simulink model "sobelFilter2024a"  (R2024b)
settings: Solver=FixedStepDiscrete  StartTime=0.0  StopTime=2  FixedStep=1/(R*C)  RelTol=1e-3
undefined symbols (not defined in the file or in its folder): gray, R
libraries: hdlsllib x13, visionhdlio x4, visionsources x2
(part 2 of 2)

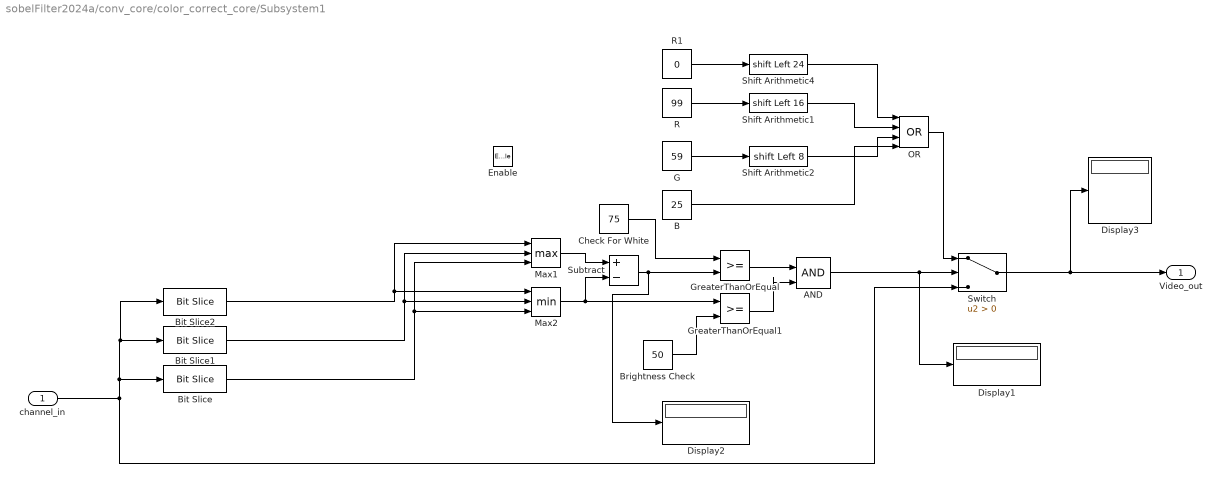
== system sobelFilter2024a/conv_core/color_correct_core/Subsystem1 ==
  channel_in : Inport  OutDataTypeStr=uint32
  Enable : EnablePort
  AND : Logic  IconShape=distinctive  AllPortsSameDT=off  OutDataTypeStr=boolean
  B : Constant  Value=25  OutDataTypeStr=uint8
  Bit Slice : hdlsllib/Logic and Bit Operations/Bit Slice  lidx=7  ridx=0
  Bit Slice1 : hdlsllib/Logic and Bit Operations/Bit Slice  lidx=15  ridx=8
  Bit Slice2 : hdlsllib/Logic and Bit Operations/Bit Slice  lidx=23  ridx=16
  Brightness Check : Constant  Value=50  OutDataTypeStr=uint8
  Check For White : Constant  Value=75  OutDataTypeStr=uint8
  Display1 : Display
      settings: Format=binary (Stored Integer)
  Display2 : Display
      settings: Format=binary (Stored Integer)
  Display3 : Display
      settings: Format=binary (Stored Integer)
  G : Constant  Value=59  OutDataTypeStr=uint8
  GreaterThanOrEqual : RelationalOperator  OutDataTypeStr=boolean  RndMeth=Simplest  InputSameDT=off
  GreaterThanOrEqual1 : RelationalOperator  OutDataTypeStr=boolean  RndMeth=Simplest  InputSameDT=off
  Max1 : MinMax  Function=max  Inputs=3  OutDataTypeStr=uint8
  Max2 : MinMax  Inputs=3  OutDataTypeStr=uint8
  OR : Logic  Operator=OR  Inputs=4  IconShape=distinctive  AllPortsSameDT=off
  R : Constant  Value=99  OutDataTypeStr=uint8
  R1 : Constant  Value=0  OutDataTypeStr=uint8
  Shift Arithmetic1 : ArithShift  BitShiftNumber=16  BitShiftDirection=Left
  Shift Arithmetic2 : ArithShift  BitShiftNumber=8  BitShiftDirection=Left
  Shift Arithmetic4 : ArithShift  BitShiftNumber=24  BitShiftDirection=Left
  Subtract : Sum  Inputs=+-
  Switch : Switch  Criteria=u2 > Threshold  OutDataTypeStr=uint32  SaturateOnIntegerOverflow=off  InputSameDT=off
  Video_out : Outport  OutDataTypeStr=uint32  InitialOutput=[0]
  wires:
  channel_in/1 -> Switch/3, Bit Slice2/1, Bit Slice1/1, Bit Slice/1
  Max1/1 -> Subtract/1
  Max2/1 -> GreaterThanOrEqual1/1, Subtract/2
  Check For White/1 -> GreaterThanOrEqual/1
  GreaterThanOrEqual/1 -> AND/1
  Brightness Check/1 -> GreaterThanOrEqual1/2
  GreaterThanOrEqual1/1 -> AND/2
  Subtract/1 -> GreaterThanOrEqual/2, Display2/1
  AND/1 -> Display1/1, Switch/2
  Switch/1 -> Display3/1, Video_out/1
  Bit Slice2/1 -> Max1/1, Max2/1
  Bit Slice1/1 -> Max2/2, Max1/2
  Bit Slice/1 -> Max2/3, Max1/3
  R1/1 -> Shift Arithmetic4/1
  R/1 -> Shift Arithmetic1/1
  G/1 -> Shift Arithmetic2/1
  B/1 -> OR/4
  Shift Arithmetic2/1 -> OR/3
  Shift Arithmetic1/1 -> OR/2
  Shift Arithmetic4/1 -> OR/1
  OR/1 -> Switch/1

== system sobelFilter2024a/conv_core/gaussian_conv_core/Subsystem1 ==
  note: slice out gray
  channel_in : Inport  OutDataTypeStr=uint8
  coeffs : Inport  Port=2
  Enable : EnablePort
  Delay1 : Delay  DelayLength=1  InitialCondition=0
  Delay2 : Delay  DelayLength=1  InitialCondition=0
  Display : Display
      settings: Format=hex (Stored Integer)
  Mux : Mux  Inputs=9
  Product : Product  SaturateOnIntegerOverflow=on
  Sum of Elements : Sum  Inputs=+  OutDataTypeStr=uint8  SaturateOnIntegerOverflow=on
  slicer : Subsystem
  Video_out : Outport  OutDataTypeStr=uint8  InitialOutput=[0]
  wires:
  slicer/1(out_1) -> Mux/1
  slicer/9(out_9) -> Mux/9
  slicer/5(out_5) -> Mux/5
  slicer/7(out_7) -> Mux/7
  slicer/3(out_3) -> Mux/3
  slicer/6(out_6) -> Mux/6
  slicer/4(out_4) -> Mux/4
  slicer/2(out_2) -> Mux/2
  channel_in/1 -> slicer/1(channel_in)
  slicer/8(out_8) -> Mux/8
  Mux/1 -> Product/2
  coeffs/1 -> Product/1, Display/1
  Product/1 -> Delay1/1
  Delay1/1 -> Sum of Elements/1
  Sum of Elements/1 -> Delay2/1
  Delay2/1 -> Video_out/1

== system sobelFilter2024a/conv_core/just_gray_core/Subsystem1 ==
  note: slice out gray
  note: Grayscale = (R * 0.25) + (G * 0.5) + (B * 0.0625)
  channel_in : Inport  OutDataTypeStr=uint32
  Enable : EnablePort
  Bit Slice1 : hdlsllib/Logic and Bit Operations/Bit Slice  lidx=7  ridx=0
  Bit Slice2 : hdlsllib/Logic and Bit Operations/Bit Slice  lidx=15  ridx=8
  Bit Slice3 : hdlsllib/Logic and Bit Operations/Bit Slice  lidx=23  ridx=16
  Shift Arithmetic3 : ArithShift  BitShiftNumber=1  BitShiftDirection=Right
  Shift Arithmetic4 : ArithShift  BitShiftNumber=2  BitShiftDirection=Right
  Shift Arithmetic5 : ArithShift  BitShiftNumber=4  BitShiftDirection=Right
  Sum : Sum  Inputs=+++  OutDataTypeStr=uint8
  Video_out : Outport  OutDataTypeStr=uint8  InitialOutput=[0]
  wires:
  Shift Arithmetic4/1 -> Sum/1
  Shift Arithmetic3/1 -> Sum/2
  Shift Arithmetic5/1 -> Sum/3
  Bit Slice2/1 -> Shift Arithmetic3/1
  Bit Slice3/1 -> Shift Arithmetic4/1
  channel_in/1 -> Bit Slice3/1, Bit Slice2/1, Bit Slice1/1
  Sum/1 -> Video_out/1
  Bit Slice1/1 -> Shift Arithmetic5/1

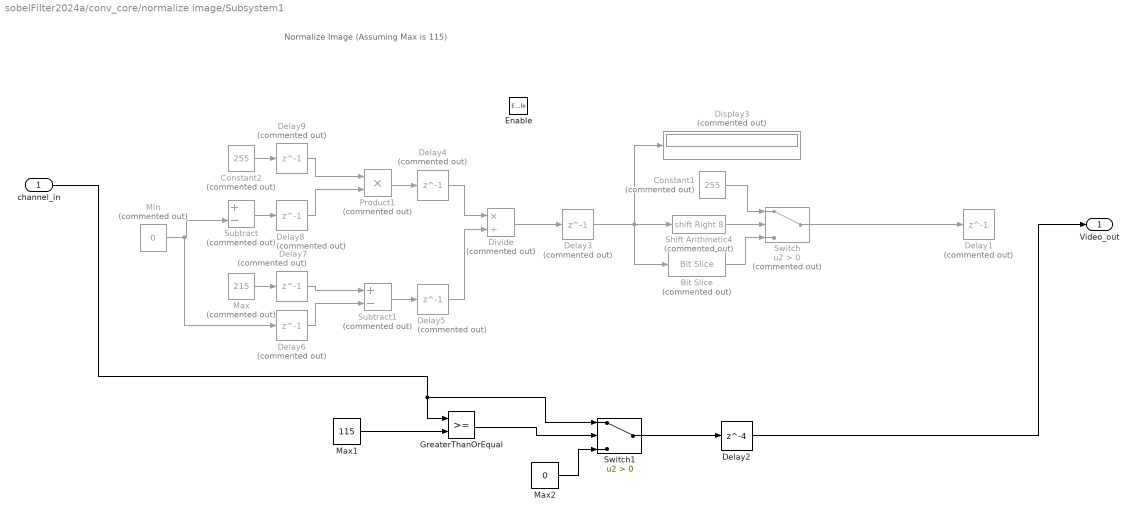
== system sobelFilter2024a/conv_core/normalize image/Subsystem1 ==
  note: Normalize Image (Assuming Max is 115)
  channel_in : Inport  OutDataTypeStr=uint8
  Enable : EnablePort
  Bit Slice : hdlsllib/Logic and Bit Operations/Bit Slice  Commented=on  lidx=7  ridx=0
  Constant1 : Constant  Commented=on  Value=255  OutDataTypeStr=uint8
  Constant2 : Constant  Commented=on  Value=255  OutDataTypeStr=uint8
  Delay{1,3..9} (8 alike) : Delay  Commented=on  DelayLength=1  InitialCondition=0
  Delay2 : Delay  DelayLength=4  InitialCondition=0
  Display3 : Display  Commented=on
      settings: Format=binary (Stored Integer)
  Divide : Product  Commented=on  Inputs=*/
  GreaterThanOrEqual : RelationalOperator  OutDataTypeStr=boolean  RndMeth=Simplest  InputSameDT=off
  Max : Constant  Commented=on  Value=215  OutDataTypeStr=uint8
  Max1 : Constant  Value=115  OutDataTypeStr=uint8
  Max2 : Constant  Value=0  OutDataTypeStr=uint8
  Min : Constant  Commented=on  Value=0  OutDataTypeStr=uint8
  Product1 : Product  Commented=on  SaturateOnIntegerOverflow=on
  Shift Arithmetic4 : ArithShift  Commented=on  BitShiftNumber=8  BitShiftDirection=Right
  Subtract : Sum  Commented=on  Inputs=+-  AccumDataTypeStr=uint8
  Subtract1 : Sum  Commented=on  Inputs=+-  OutDataTypeStr=uint8
  Switch : Switch  Commented=on  Criteria=u2 > Threshold  SaturateOnIntegerOverflow=off  InputSameDT=off
  Switch1 : Switch  Criteria=u2 > Threshold  SaturateOnIntegerOverflow=off  InputSameDT=off
  Video_out : Outport  OutDataTypeStr=uint8  InitialOutput=[0]
  wires:
  Constant2/1 -> Delay9/1
  Subtract/1 -> Delay8/1
  Product1/1 -> Delay4/1
  Max/1 -> Delay7/1
  Min/1 -> Delay6/1, Subtract/2
  Subtract1/1 -> Delay5/1
  Divide/1 -> Delay3/1
  Delay3/1 -> Bit Slice/1, Shift Arithmetic4/1, Display3/1
  Delay4/1 -> Divide/1
  Delay5/1 -> Divide/2
  Delay6/1 -> Subtract1/2
  Delay7/1 -> Subtract1/1
  Delay8/1 -> Product1/2
  Delay9/1 -> Product1/1
  Shift Arithmetic4/1 -> Switch/2
  Switch/1 -> Delay1/1
  Constant1/1 -> Switch/1
  Bit Slice/1 -> Switch/3
  Max1/1 -> GreaterThanOrEqual/2
  channel_in/1 -> Switch1/1, GreaterThanOrEqual/1
  GreaterThanOrEqual/1 -> Switch1/2
  Max2/1 -> Switch1/3
  Switch1/1 -> Delay2/1
  Delay2/1 -> Video_out/1

== system sobelFilter2024a/conv_core/sobel_horz_conv_core/Subsystem1 ==
  note: slice out gray
  channel_in : Inport  OutDataTypeStr=uint8
  coeffs : Inport  Port=2
  Enable : EnablePort
  Delay1 : Delay  DelayLength=1  InitialCondition=0
  Delay2 : Delay  DelayLength=1  InitialCondition=0
  Display : Display
      settings: Format=hex (Stored Integer)
  Mux : Mux  Inputs=9
  Product : Product  SaturateOnIntegerOverflow=on
  Sum of Elements : Sum  Inputs=+  OutDataTypeStr=uint8  SaturateOnIntegerOverflow=on
  slicer : Subsystem
  Video_out : Outport  OutDataTypeStr=uint8  InitialOutput=[0]
  wires:
  slicer/1(out_1) -> Mux/1
  slicer/9(out_9) -> Mux/9
  slicer/5(out_5) -> Mux/5
  slicer/7(out_7) -> Mux/7
  slicer/3(out_3) -> Mux/3
  slicer/6(out_6) -> Mux/6
  slicer/4(out_4) -> Mux/4
  slicer/2(out_2) -> Mux/2
  channel_in/1 -> slicer/1(channel_in)
  slicer/8(out_8) -> Mux/8
  Mux/1 -> Product/2
  coeffs/1 -> Product/1, Display/1
  Product/1 -> Delay1/1
  Delay1/1 -> Sum of Elements/1
  Sum of Elements/1 -> Delay2/1
  Delay2/1 -> Video_out/1

== system sobelFilter2024a/conv_core/sobel_horz_conv_core_alt/Subsystem1 ==
  note: slice out gray
  channel_in : Inport  OutDataTypeStr=uint8
  coeffs : Inport  Port=2
  Enable : EnablePort
  Delay1 : Delay  DelayLength=1  InitialCondition=0
  Delay2 : Delay  DelayLength=1  InitialCondition=0
  Display : Display
      settings: Format=hex (Stored Integer)
  Mux : Mux  Inputs=9
  Product : Product  SaturateOnIntegerOverflow=on
  Sum of Elements : Sum  Inputs=+  OutDataTypeStr=uint8  SaturateOnIntegerOverflow=on
  slicer : Subsystem
  Video_out : Outport  OutDataTypeStr=uint8  InitialOutput=[0]
  wires:
  slicer/1(out_1) -> Mux/1
  slicer/9(out_9) -> Mux/9
  slicer/5(out_5) -> Mux/5
  slicer/7(out_7) -> Mux/7
  slicer/3(out_3) -> Mux/3
  slicer/6(out_6) -> Mux/6
  slicer/4(out_4) -> Mux/4
  slicer/2(out_2) -> Mux/2
  channel_in/1 -> slicer/1(channel_in)
  slicer/8(out_8) -> Mux/8
  Mux/1 -> Product/2
  coeffs/1 -> Product/1, Display/1
  Product/1 -> Delay1/1
  Delay1/1 -> Sum of Elements/1
  Sum of Elements/1 -> Delay2/1
  Delay2/1 -> Video_out/1

== system sobelFilter2024a/conv_core/sobel_vert_conv_core/Subsystem1 ==
  note: slice out gray
  channel_in : Inport  OutDataTypeStr=uint8
  coeffs : Inport  Port=2
  Enable : EnablePort
  Delay1 : Delay  DelayLength=1  InitialCondition=0
  Delay2 : Delay  DelayLength=1  InitialCondition=0
  Display : Display
      settings: Format=hex (Stored Integer)
  Mux : Mux  Inputs=9
  Product : Product  SaturateOnIntegerOverflow=on
  Sum of Elements : Sum  Inputs=+  OutDataTypeStr=uint8  SaturateOnIntegerOverflow=on
  slicer : Subsystem
  Video_out : Outport  OutDataTypeStr=uint8  InitialOutput=[0]
  wires:
  slicer/1(out_1) -> Mux/1
  slicer/9(out_9) -> Mux/9
  slicer/5(out_5) -> Mux/5
  slicer/7(out_7) -> Mux/7
  slicer/3(out_3) -> Mux/3
  slicer/6(out_6) -> Mux/6
  slicer/4(out_4) -> Mux/4
  slicer/2(out_2) -> Mux/2
  channel_in/1 -> slicer/1(channel_in)
  slicer/8(out_8) -> Mux/8
  Mux/1 -> Product/2
  coeffs/1 -> Product/1, Display/1
  Product/1 -> Delay1/1
  Delay1/1 -> Sum of Elements/1
  Sum of Elements/1 -> Delay2/1
  Delay2/1 -> Video_out/1

== system sobelFilter2024a/conv_core/sobel_vert_conv_core_alt/Subsystem1 ==
  note: slice out gray
  channel_in : Inport  OutDataTypeStr=uint8
  coeffs : Inport  Port=2
  Enable : EnablePort
  Delay1 : Delay  DelayLength=1  InitialCondition=0
  Delay2 : Delay  DelayLength=1  InitialCondition=0
  Display : Display
      settings: Format=hex (Stored Integer)
  Mux : Mux  Inputs=9
  Product : Product  SaturateOnIntegerOverflow=on
  Sum of Elements : Sum  Inputs=+  OutDataTypeStr=uint8  SaturateOnIntegerOverflow=on
  slicer : Subsystem
  Video_out : Outport  OutDataTypeStr=uint8  InitialOutput=[0]
  wires:
  slicer/1(out_1) -> Mux/1
  slicer/9(out_9) -> Mux/9
  slicer/5(out_5) -> Mux/5
  slicer/7(out_7) -> Mux/7
  slicer/3(out_3) -> Mux/3
  slicer/6(out_6) -> Mux/6
  slicer/4(out_4) -> Mux/4
  slicer/2(out_2) -> Mux/2
  channel_in/1 -> slicer/1(channel_in)
  slicer/8(out_8) -> Mux/8
  Mux/1 -> Product/2
  coeffs/1 -> Product/1, Display/1
  Product/1 -> Delay1/1
  Delay1/1 -> Sum of Elements/1
  Sum of Elements/1 -> Delay2/1
  Delay2/1 -> Video_out/1

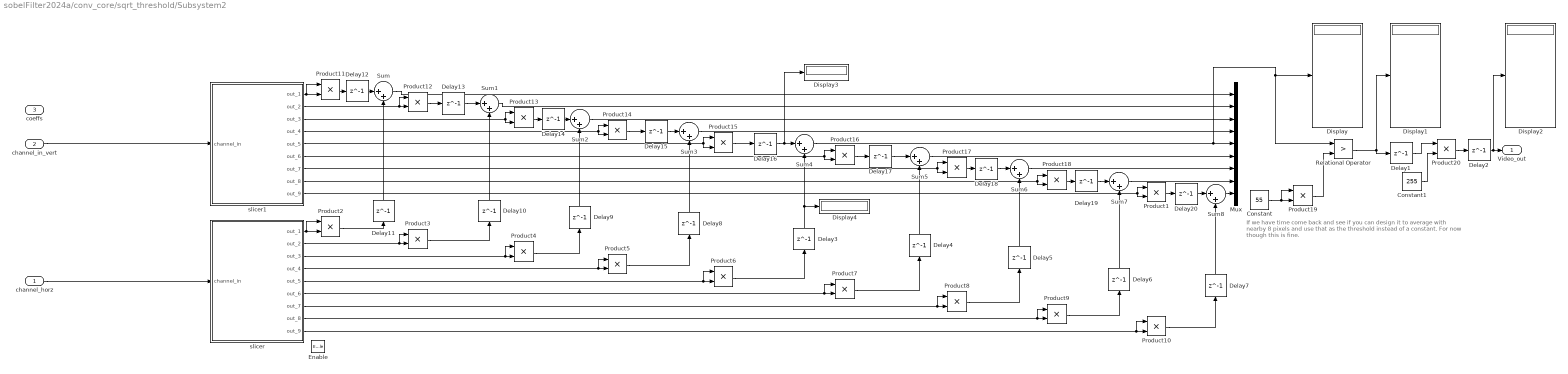
== system sobelFilter2024a/conv_core/sqrt_threshold/Subsystem2 ==
  note: If we have time come back and see if you can design it to average with
      | nearby 8 pixels and use that as the threshold instead of a constant. For
      |  now though this is fine.
  channel_horz : Inport  OutDataTypeStr=uint8
  channel_in_vert : Inport  Port=2
  coeffs : Inport  Port=3
  Enable : EnablePort
  Constant : Constant  Value=55  OutDataTypeStr=uint8
  Constant1 : Constant  Value=255  OutDataTypeStr=uint8
  Delay{1..20} (20 alike) : Delay  DelayLength=1  InitialCondition=0
  Display{,1..4} (5 alike) : Display
      settings: Format=decimal (Stored Integer)
  Mux : Mux  Inputs=9
  Product{1..20} (20 alike) : Product  SaturateOnIntegerOverflow=on
  Relational Operator : RelationalOperator  Operator=>  OutDataTypeStr=boolean  InputSameDT=off
  Sum{,1..8} (9 alike) : Sum  Inputs=|++
  slicer : Subsystem
  slicer1 : Subsystem
  Video_out : Outport  OutDataTypeStr=uint8  InitialOutput=[0]
  wires:
  slicer/1(out_1) -> Product2/1, Product2/2
  slicer/5(out_5) -> Product6/1, Product6/2
  slicer/7(out_7) -> Product8/1, Product8/2
  slicer/3(out_3) -> Product4/1, Product4/2
  slicer/6(out_6) -> Product7/1, Product7/2
  slicer/4(out_4) -> Product5/1, Product5/2
  slicer/2(out_2) -> Product3/1, Product3/2
  channel_horz/1 -> slicer/1(channel_in)
  slicer/8(out_8) -> Product9/1, Product9/2
  Delay2/1 -> Display2/1, Video_out/1
  slicer/9(out_9) -> Product10/1, Product10/2
  slicer1/8(out_8) -> Product18/2, Product18/1
  slicer1/2(out_2) -> Product12/1, Product12/2
  slicer1/9(out_9) -> Product1/2, Product1/1
  slicer1/1(out_1) -> Product11/1, Product11/2
  slicer1/3(out_3) -> Product13/2, Product13/1
  slicer1/7(out_7) -> Product17/2, Product17/1
  slicer1/5(out_5) -> Product15/2, Product15/1
  slicer1/6(out_6) -> Product16/2, Product16/1
  slicer1/4(out_4) -> Product14/2, Product14/1
  channel_in_vert/1 -> slicer1/1(channel_in)
  Product2/1 -> Delay11/1
  Product12/1 -> Delay13/1
  Product3/1 -> Delay10/1
  Product4/1 -> Delay9/1
  Product14/1 -> Delay15/1
  Product5/1 -> Delay8/1
  Product15/1 -> Delay16/1
  Product6/1 -> Delay3/1
  Product16/1 -> Delay17/1
  Product7/1 -> Delay4/1
  Product8/1 -> Delay5/1
  Product9/1 -> Delay6/1
  Product10/1 -> Delay7/1
  Delay1/1 -> Product20/1
  Delay3/1 -> Display4/1, Sum4/2
  Delay4/1 -> Sum5/2
  Delay5/1 -> Sum6/2
  Delay6/1 -> Sum7/2
  Delay7/1 -> Sum8/2
  Delay8/1 -> Sum3/2
  Delay9/1 -> Sum2/2
  Delay10/1 -> Sum1/2
  Delay11/1 -> Sum/2
  Product11/1 -> Delay12/1
  Delay12/1 -> Sum/1
  Delay13/1 -> Sum1/1
  Product13/1 -> Delay14/1
  Delay14/1 -> Sum2/1
  Delay15/1 -> Sum3/1
  Delay16/1 -> Display3/1, Sum4/1
  Delay17/1 -> Sum5/1
  Product17/1 -> Delay18/1
  Delay18/1 -> Sum6/1
  Product18/1 -> Delay19/1
  Delay19/1 -> Sum7/1
  Product1/1 -> Delay20/1
  Delay20/1 -> Sum8/1
  Sum8/1 -> Mux/9
  Sum7/1 -> Mux/8
  Sum6/1 -> Mux/7
  Sum5/1 -> Mux/6
  Sum3/1 -> Mux/4
  Sum2/1 -> Mux/3
  Sum1/1 -> Mux/2
  Sum/1 -> Mux/1
  Constant/1 -> Product19/1, Product19/2
  Product19/1 -> Relational Operator/2
  Relational Operator/1 -> Display1/1, Delay1/1
  Sum4/1 -> Display/1, Relational Operator/1, Mux/5
  Constant1/1 -> Product20/2
  Product20/1 -> Delay2/1

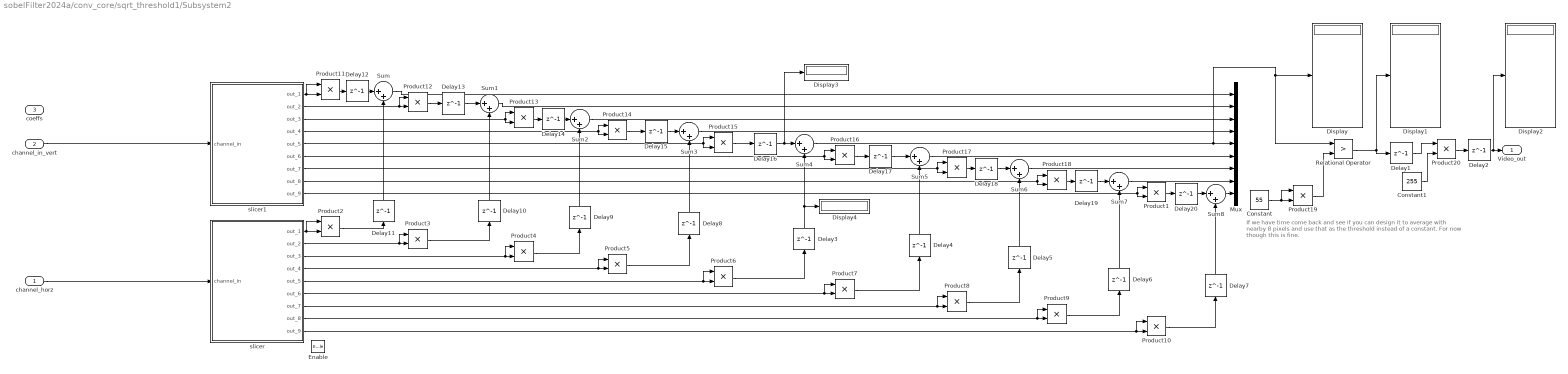
== system sobelFilter2024a/conv_core/sqrt_threshold1/Subsystem2 ==
  note: If we have time come back and see if you can design it to average with
      | nearby 8 pixels and use that as the threshold instead of a constant. For
      |  now though this is fine.
  channel_horz : Inport  OutDataTypeStr=uint8
  channel_in_vert : Inport  Port=2
  coeffs : Inport  Port=3
  Enable : EnablePort
  Constant : Constant  Value=55  OutDataTypeStr=uint8
  Constant1 : Constant  Value=255  OutDataTypeStr=uint8
  Delay{1..20} (20 alike) : Delay  DelayLength=1  InitialCondition=0
  Display{,1..4} (5 alike) : Display
      settings: Format=decimal (Stored Integer)
  Mux : Mux  Inputs=9
  Product{1..20} (20 alike) : Product  SaturateOnIntegerOverflow=on
  Relational Operator : RelationalOperator  Operator=>  OutDataTypeStr=boolean  InputSameDT=off
  Sum{,1..8} (9 alike) : Sum  Inputs=|++
  slicer : Subsystem
  slicer1 : Subsystem
  Video_out : Outport  OutDataTypeStr=uint8  InitialOutput=[0]
  wires:
  slicer/1(out_1) -> Product2/1, Product2/2
  slicer/5(out_5) -> Product6/1, Product6/2
  slicer/7(out_7) -> Product8/1, Product8/2
  slicer/3(out_3) -> Product4/1, Product4/2
  slicer/6(out_6) -> Product7/1, Product7/2
  slicer/4(out_4) -> Product5/1, Product5/2
  slicer/2(out_2) -> Product3/1, Product3/2
  channel_horz/1 -> slicer/1(channel_in)
  slicer/8(out_8) -> Product9/1, Product9/2
  Delay2/1 -> Display2/1, Video_out/1
  slicer/9(out_9) -> Product10/1, Product10/2
  slicer1/8(out_8) -> Product18/2, Product18/1
  slicer1/2(out_2) -> Product12/1, Product12/2
  slicer1/9(out_9) -> Product1/2, Product1/1
  slicer1/1(out_1) -> Product11/1, Product11/2
  slicer1/3(out_3) -> Product13/2, Product13/1
  slicer1/7(out_7) -> Product17/2, Product17/1
  slicer1/5(out_5) -> Product15/2, Product15/1
  slicer1/6(out_6) -> Product16/2, Product16/1
  slicer1/4(out_4) -> Product14/2, Product14/1
  channel_in_vert/1 -> slicer1/1(channel_in)
  Product2/1 -> Delay11/1
  Product12/1 -> Delay13/1
  Product3/1 -> Delay10/1
  Product4/1 -> Delay9/1
  Product14/1 -> Delay15/1
  Product5/1 -> Delay8/1
  Product15/1 -> Delay16/1
  Product6/1 -> Delay3/1
  Product16/1 -> Delay17/1
  Product7/1 -> Delay4/1
  Product8/1 -> Delay5/1
  Product9/1 -> Delay6/1
  Product10/1 -> Delay7/1
  Delay1/1 -> Product20/1
  Delay3/1 -> Display4/1, Sum4/2
  Delay4/1 -> Sum5/2
  Delay5/1 -> Sum6/2
  Delay6/1 -> Sum7/2
  Delay7/1 -> Sum8/2
  Delay8/1 -> Sum3/2
  Delay9/1 -> Sum2/2
  Delay10/1 -> Sum1/2
  Delay11/1 -> Sum/2
  Product11/1 -> Delay12/1
  Delay12/1 -> Sum/1
  Delay13/1 -> Sum1/1
  Product13/1 -> Delay14/1
  Delay14/1 -> Sum2/1
  Delay15/1 -> Sum3/1
  Delay16/1 -> Display3/1, Sum4/1
  Delay17/1 -> Sum5/1
  Product17/1 -> Delay18/1
  Delay18/1 -> Sum6/1
  Product18/1 -> Delay19/1
  Delay19/1 -> Sum7/1
  Product1/1 -> Delay20/1
  Delay20/1 -> Sum8/1
  Sum8/1 -> Mux/9
  Sum7/1 -> Mux/8
  Sum6/1 -> Mux/7
  Sum5/1 -> Mux/6
  Sum3/1 -> Mux/4
  Sum2/1 -> Mux/3
  Sum1/1 -> Mux/2
  Sum/1 -> Mux/1
  Constant/1 -> Product19/1, Product19/2
  Product19/1 -> Relational Operator/2
  Relational Operator/1 -> Display1/1, Delay1/1
  Sum4/1 -> Display/1, Relational Operator/1, Mux/5
  Constant1/1 -> Product20/2
  Product20/1 -> Delay2/1

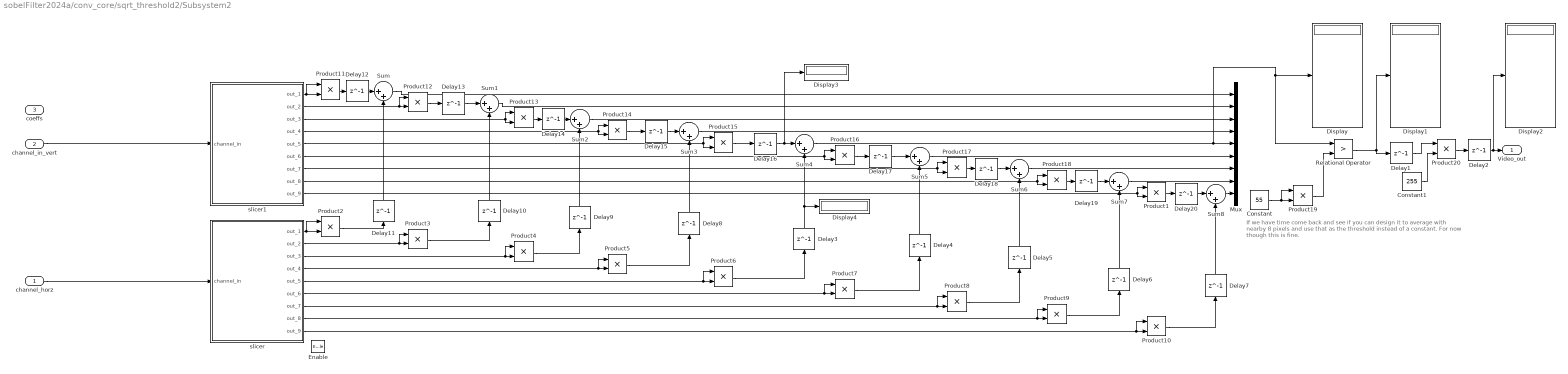
== system sobelFilter2024a/conv_core/sqrt_threshold2/Subsystem2 ==
  note: If we have time come back and see if you can design it to average with
      | nearby 8 pixels and use that as the threshold instead of a constant. For
      |  now though this is fine.
  channel_horz : Inport  OutDataTypeStr=uint8
  channel_in_vert : Inport  Port=2
  coeffs : Inport  Port=3
  Enable : EnablePort
  Constant : Constant  Value=55  OutDataTypeStr=uint8
  Constant1 : Constant  Value=255  OutDataTypeStr=uint8
  Delay{1..20} (20 alike) : Delay  DelayLength=1  InitialCondition=0
  Display{,1..4} (5 alike) : Display
      settings: Format=decimal (Stored Integer)
  Mux : Mux  Inputs=9
  Product{1..20} (20 alike) : Product  SaturateOnIntegerOverflow=on
  Relational Operator : RelationalOperator  Operator=>  OutDataTypeStr=boolean  InputSameDT=off
  Sum{,1..8} (9 alike) : Sum  Inputs=|++
  slicer : Subsystem
  slicer1 : Subsystem
  Video_out : Outport  OutDataTypeStr=uint8  InitialOutput=[0]
  wires:
  slicer/1(out_1) -> Product2/1, Product2/2
  slicer/5(out_5) -> Product6/1, Product6/2
  slicer/7(out_7) -> Product8/1, Product8/2
  slicer/3(out_3) -> Product4/1, Product4/2
  slicer/6(out_6) -> Product7/1, Product7/2
  slicer/4(out_4) -> Product5/1, Product5/2
  slicer/2(out_2) -> Product3/1, Product3/2
  channel_horz/1 -> slicer/1(channel_in)
  slicer/8(out_8) -> Product9/1, Product9/2
  Delay2/1 -> Display2/1, Video_out/1
  slicer/9(out_9) -> Product10/1, Product10/2
  slicer1/8(out_8) -> Product18/2, Product18/1
  slicer1/2(out_2) -> Product12/1, Product12/2
  slicer1/9(out_9) -> Product1/2, Product1/1
  slicer1/1(out_1) -> Product11/1, Product11/2
  slicer1/3(out_3) -> Product13/2, Product13/1
  slicer1/7(out_7) -> Product17/2, Product17/1
  slicer1/5(out_5) -> Product15/2, Product15/1
  slicer1/6(out_6) -> Product16/2, Product16/1
  slicer1/4(out_4) -> Product14/2, Product14/1
  channel_in_vert/1 -> slicer1/1(channel_in)
  Product2/1 -> Delay11/1
  Product12/1 -> Delay13/1
  Product3/1 -> Delay10/1
  Product4/1 -> Delay9/1
  Product14/1 -> Delay15/1
  Product5/1 -> Delay8/1
  Product15/1 -> Delay16/1
  Product6/1 -> Delay3/1
  Product16/1 -> Delay17/1
  Product7/1 -> Delay4/1
  Product8/1 -> Delay5/1
  Product9/1 -> Delay6/1
  Product10/1 -> Delay7/1
  Delay1/1 -> Product20/1
  Delay3/1 -> Display4/1, Sum4/2
  Delay4/1 -> Sum5/2
  Delay5/1 -> Sum6/2
  Delay6/1 -> Sum7/2
  Delay7/1 -> Sum8/2
  Delay8/1 -> Sum3/2
  Delay9/1 -> Sum2/2
  Delay10/1 -> Sum1/2
  Delay11/1 -> Sum/2
  Product11/1 -> Delay12/1
  Delay12/1 -> Sum/1
  Delay13/1 -> Sum1/1
  Product13/1 -> Delay14/1
  Delay14/1 -> Sum2/1
  Delay15/1 -> Sum3/1
  Delay16/1 -> Display3/1, Sum4/1
  Delay17/1 -> Sum5/1
  Product17/1 -> Delay18/1
  Delay18/1 -> Sum6/1
  Product18/1 -> Delay19/1
  Delay19/1 -> Sum7/1
  Product1/1 -> Delay20/1
  Delay20/1 -> Sum8/1
  Sum8/1 -> Mux/9
  Sum7/1 -> Mux/8
  Sum6/1 -> Mux/7
  Sum5/1 -> Mux/6
  Sum3/1 -> Mux/4
  Sum2/1 -> Mux/3
  Sum1/1 -> Mux/2
  Sum/1 -> Mux/1
  Constant/1 -> Product19/1, Product19/2
  Product19/1 -> Relational Operator/2
  Relational Operator/1 -> Display1/1, Delay1/1
  Sum4/1 -> Display/1, Relational Operator/1, Mux/5
  Constant1/1 -> Product20/2
  Product20/1 -> Delay2/1

== system sobelFilter2024a/gaussian_conv_core/Subsystem1/slicer ==
  channel_in : Inport
  Delay{1..6} (6 alike) : Delay  DelayLength=1  InitialCondition=0
  Line buffer : Delay  DelayLength=R-2  InitialCondition=0
  Line buffer1 : Delay  DelayLength=R-2  InitialCondition=0
  out_1 : Outport  VectorParamsAs1DForOutWhenUnconnected=off
  out_2 : Outport  Port=2  VectorParamsAs1DForOutWhenUnconnected=off
  out_3 : Outport  Port=3  VectorParamsAs1DForOutWhenUnconnected=off
  out_4 : Outport  Port=4  VectorParamsAs1DForOutWhenUnconnected=off
  out_5 : Outport  Port=5  VectorParamsAs1DForOutWhenUnconnected=off
  out_6 : Outport  Port=6  VectorParamsAs1DForOutWhenUnconnected=off
  out_7 : Outport  Port=7  VectorParamsAs1DForOutWhenUnconnected=off
  out_8 : Outport  Port=8  VectorParamsAs1DForOutWhenUnconnected=off
  out_9 : Outport  Port=9  VectorParamsAs1DForOutWhenUnconnected=off
  wires:
  Delay4/1 -> Line buffer/1, out_3/1
  channel_in/1 -> out_1/1, Delay1/1
  Delay1/1 -> out_2/1, Delay4/1
  Delay3/1 -> out_8/1, Delay6/1
  Delay5/1 -> Line buffer1/1, out_6/1
  Delay6/1 -> out_9/1
  Line buffer/1 -> out_4/1, Delay2/1
  Line buffer1/1 -> out_7/1, Delay3/1
  Delay2/1 -> out_5/1, Delay5/1

== system sobelFilter2024a/sobel_horz_conv_core/Subsystem1/slicer ==
  channel_in : Inport
  Delay{1..6} (6 alike) : Delay  DelayLength=1  InitialCondition=0
  Line buffer : Delay  DelayLength=R-2  InitialCondition=0
  Line buffer1 : Delay  DelayLength=R-2  InitialCondition=0
  out_1 : Outport  VectorParamsAs1DForOutWhenUnconnected=off
  out_2 : Outport  Port=2  VectorParamsAs1DForOutWhenUnconnected=off
  out_3 : Outport  Port=3  VectorParamsAs1DForOutWhenUnconnected=off
  out_4 : Outport  Port=4  VectorParamsAs1DForOutWhenUnconnected=off
  out_5 : Outport  Port=5  VectorParamsAs1DForOutWhenUnconnected=off
  out_6 : Outport  Port=6  VectorParamsAs1DForOutWhenUnconnected=off
  out_7 : Outport  Port=7  VectorParamsAs1DForOutWhenUnconnected=off
  out_8 : Outport  Port=8  VectorParamsAs1DForOutWhenUnconnected=off
  out_9 : Outport  Port=9  VectorParamsAs1DForOutWhenUnconnected=off
  wires:
  Delay4/1 -> Line buffer/1, out_3/1
  channel_in/1 -> out_1/1, Delay1/1
  Delay1/1 -> out_2/1, Delay4/1
  Delay3/1 -> out_8/1, Delay6/1
  Delay5/1 -> Line buffer1/1, out_6/1
  Delay6/1 -> out_9/1
  Line buffer/1 -> out_4/1, Delay2/1
  Line buffer1/1 -> out_7/1, Delay3/1
  Delay2/1 -> out_5/1, Delay5/1

== system sobelFilter2024a/sobel_horz_conv_core_alt/Subsystem1/slicer ==
  channel_in : Inport
  Delay{1..6} (6 alike) : Delay  DelayLength=1  InitialCondition=0
  Line buffer : Delay  DelayLength=R-2  InitialCondition=0
  Line buffer1 : Delay  DelayLength=R-2  InitialCondition=0
  out_1 : Outport  VectorParamsAs1DForOutWhenUnconnected=off
  out_2 : Outport  Port=2  VectorParamsAs1DForOutWhenUnconnected=off
  out_3 : Outport  Port=3  VectorParamsAs1DForOutWhenUnconnected=off
  out_4 : Outport  Port=4  VectorParamsAs1DForOutWhenUnconnected=off
  out_5 : Outport  Port=5  VectorParamsAs1DForOutWhenUnconnected=off
  out_6 : Outport  Port=6  VectorParamsAs1DForOutWhenUnconnected=off
  out_7 : Outport  Port=7  VectorParamsAs1DForOutWhenUnconnected=off
  out_8 : Outport  Port=8  VectorParamsAs1DForOutWhenUnconnected=off
  out_9 : Outport  Port=9  VectorParamsAs1DForOutWhenUnconnected=off
  wires:
  Delay4/1 -> Line buffer/1, out_3/1
  channel_in/1 -> out_1/1, Delay1/1
  Delay1/1 -> out_2/1, Delay4/1
  Delay3/1 -> out_8/1, Delay6/1
  Delay5/1 -> Line buffer1/1, out_6/1
  Delay6/1 -> out_9/1
  Line buffer/1 -> out_4/1, Delay2/1
  Line buffer1/1 -> out_7/1, Delay3/1
  Delay2/1 -> out_5/1, Delay5/1

== system sobelFilter2024a/sobel_vert_conv_core/Subsystem1/slicer ==
  channel_in : Inport
  Delay{1..6} (6 alike) : Delay  DelayLength=1  InitialCondition=0
  Line buffer : Delay  DelayLength=R-2  InitialCondition=0
  Line buffer1 : Delay  DelayLength=R-2  InitialCondition=0
  out_1 : Outport  VectorParamsAs1DForOutWhenUnconnected=off
  out_2 : Outport  Port=2  VectorParamsAs1DForOutWhenUnconnected=off
  out_3 : Outport  Port=3  VectorParamsAs1DForOutWhenUnconnected=off
  out_4 : Outport  Port=4  VectorParamsAs1DForOutWhenUnconnected=off
  out_5 : Outport  Port=5  VectorParamsAs1DForOutWhenUnconnected=off
  out_6 : Outport  Port=6  VectorParamsAs1DForOutWhenUnconnected=off
  out_7 : Outport  Port=7  VectorParamsAs1DForOutWhenUnconnected=off
  out_8 : Outport  Port=8  VectorParamsAs1DForOutWhenUnconnected=off
  out_9 : Outport  Port=9  VectorParamsAs1DForOutWhenUnconnected=off
  wires:
  Delay4/1 -> Line buffer/1, out_3/1
  channel_in/1 -> out_1/1, Delay1/1
  Delay1/1 -> out_2/1, Delay4/1
  Delay3/1 -> out_8/1, Delay6/1
  Delay5/1 -> Line buffer1/1, out_6/1
  Delay6/1 -> out_9/1
  Line buffer/1 -> out_4/1, Delay2/1
  Line buffer1/1 -> out_7/1, Delay3/1
  Delay2/1 -> out_5/1, Delay5/1

== system sobelFilter2024a/sobel_vert_conv_core_alt/Subsystem1/slicer ==
  channel_in : Inport
  Delay{1..6} (6 alike) : Delay  DelayLength=1  InitialCondition=0
  Line buffer : Delay  DelayLength=R-2  InitialCondition=0
  Line buffer1 : Delay  DelayLength=R-2  InitialCondition=0
  out_1 : Outport  VectorParamsAs1DForOutWhenUnconnected=off
  out_2 : Outport  Port=2  VectorParamsAs1DForOutWhenUnconnected=off
  out_3 : Outport  Port=3  VectorParamsAs1DForOutWhenUnconnected=off
  out_4 : Outport  Port=4  VectorParamsAs1DForOutWhenUnconnected=off
  out_5 : Outport  Port=5  VectorParamsAs1DForOutWhenUnconnected=off
  out_6 : Outport  Port=6  VectorParamsAs1DForOutWhenUnconnected=off
  out_7 : Outport  Port=7  VectorParamsAs1DForOutWhenUnconnected=off
  out_8 : Outport  Port=8  VectorParamsAs1DForOutWhenUnconnected=off
  out_9 : Outport  Port=9  VectorParamsAs1DForOutWhenUnconnected=off
  wires:
  Delay4/1 -> Line buffer/1, out_3/1
  channel_in/1 -> out_1/1, Delay1/1
  Delay1/1 -> out_2/1, Delay4/1
  Delay3/1 -> out_8/1, Delay6/1
  Delay5/1 -> Line buffer1/1, out_6/1
  Delay6/1 -> out_9/1
  Line buffer/1 -> out_4/1, Delay2/1
  Line buffer1/1 -> out_7/1, Delay3/1
  Delay2/1 -> out_5/1, Delay5/1

== system sobelFilter2024a/sqrt_threshold/Subsystem2/slicer ==
  channel_in : Inport
  Delay{1..6} (6 alike) : Delay  DelayLength=1  InitialCondition=0
  Line buffer : Delay  DelayLength=R-2  InitialCondition=0
  Line buffer1 : Delay  DelayLength=R-2  InitialCondition=0
  out_1 : Outport  VectorParamsAs1DForOutWhenUnconnected=off
  out_2 : Outport  Port=2  VectorParamsAs1DForOutWhenUnconnected=off
  out_3 : Outport  Port=3  VectorParamsAs1DForOutWhenUnconnected=off
  out_4 : Outport  Port=4  VectorParamsAs1DForOutWhenUnconnected=off
  out_5 : Outport  Port=5  VectorParamsAs1DForOutWhenUnconnected=off
  out_6 : Outport  Port=6  VectorParamsAs1DForOutWhenUnconnected=off
  out_7 : Outport  Port=7  VectorParamsAs1DForOutWhenUnconnected=off
  out_8 : Outport  Port=8  VectorParamsAs1DForOutWhenUnconnected=off
  out_9 : Outport  Port=9  VectorParamsAs1DForOutWhenUnconnected=off
  wires:
  Delay4/1 -> Line buffer/1, out_3/1
  channel_in/1 -> out_1/1, Delay1/1
  Delay1/1 -> out_2/1, Delay4/1
  Delay3/1 -> out_8/1, Delay6/1
  Delay5/1 -> Line buffer1/1, out_6/1
  Delay6/1 -> out_9/1
  Line buffer/1 -> out_4/1, Delay2/1
  Line buffer1/1 -> out_7/1, Delay3/1
  Delay2/1 -> out_5/1, Delay5/1

== system sobelFilter2024a/sqrt_threshold/Subsystem2/slicer1 ==
  channel_in : Inport
  Delay{1..6} (6 alike) : Delay  DelayLength=1  InitialCondition=0
  Line buffer : Delay  DelayLength=R-2  InitialCondition=0
  Line buffer1 : Delay  DelayLength=R-2  InitialCondition=0
  out_1 : Outport  VectorParamsAs1DForOutWhenUnconnected=off
  out_2 : Outport  Port=2  VectorParamsAs1DForOutWhenUnconnected=off
  out_3 : Outport  Port=3  VectorParamsAs1DForOutWhenUnconnected=off
  out_4 : Outport  Port=4  VectorParamsAs1DForOutWhenUnconnected=off
  out_5 : Outport  Port=5  VectorParamsAs1DForOutWhenUnconnected=off
  out_6 : Outport  Port=6  VectorParamsAs1DForOutWhenUnconnected=off
  out_7 : Outport  Port=7  VectorParamsAs1DForOutWhenUnconnected=off
  out_8 : Outport  Port=8  VectorParamsAs1DForOutWhenUnconnected=off
  out_9 : Outport  Port=9  VectorParamsAs1DForOutWhenUnconnected=off
  wires:
  Delay4/1 -> Line buffer/1, out_3/1
  channel_in/1 -> out_1/1, Delay1/1
  Delay1/1 -> out_2/1, Delay4/1
  Delay3/1 -> out_8/1, Delay6/1
  Delay5/1 -> Line buffer1/1, out_6/1
  Delay6/1 -> out_9/1
  Line buffer/1 -> out_4/1, Delay2/1
  Line buffer1/1 -> out_7/1, Delay3/1
  Delay2/1 -> out_5/1, Delay5/1

== system sobelFilter2024a/sqrt_threshold1/Subsystem2/slicer ==
  channel_in : Inport
  Delay{1..6} (6 alike) : Delay  DelayLength=1  InitialCondition=0
  Line buffer : Delay  DelayLength=R-2  InitialCondition=0
  Line buffer1 : Delay  DelayLength=R-2  InitialCondition=0
  out_1 : Outport  VectorParamsAs1DForOutWhenUnconnected=off
  out_2 : Outport  Port=2  VectorParamsAs1DForOutWhenUnconnected=off
  out_3 : Outport  Port=3  VectorParamsAs1DForOutWhenUnconnected=off
  out_4 : Outport  Port=4  VectorParamsAs1DForOutWhenUnconnected=off
  out_5 : Outport  Port=5  VectorParamsAs1DForOutWhenUnconnected=off
  out_6 : Outport  Port=6  VectorParamsAs1DForOutWhenUnconnected=off
  out_7 : Outport  Port=7  VectorParamsAs1DForOutWhenUnconnected=off
  out_8 : Outport  Port=8  VectorParamsAs1DForOutWhenUnconnected=off
  out_9 : Outport  Port=9  VectorParamsAs1DForOutWhenUnconnected=off
  wires:
  Delay4/1 -> Line buffer/1, out_3/1
  channel_in/1 -> out_1/1, Delay1/1
  Delay1/1 -> out_2/1, Delay4/1
  Delay3/1 -> out_8/1, Delay6/1
  Delay5/1 -> Line buffer1/1, out_6/1
  Delay6/1 -> out_9/1
  Line buffer/1 -> out_4/1, Delay2/1
  Line buffer1/1 -> out_7/1, Delay3/1
  Delay2/1 -> out_5/1, Delay5/1

== system sobelFilter2024a/sqrt_threshold1/Subsystem2/slicer1 ==
  channel_in : Inport
  Delay{1..6} (6 alike) : Delay  DelayLength=1  InitialCondition=0
  Line buffer : Delay  DelayLength=R-2  InitialCondition=0
  Line buffer1 : Delay  DelayLength=R-2  InitialCondition=0
  out_1 : Outport  VectorParamsAs1DForOutWhenUnconnected=off
  out_2 : Outport  Port=2  VectorParamsAs1DForOutWhenUnconnected=off
  out_3 : Outport  Port=3  VectorParamsAs1DForOutWhenUnconnected=off
  out_4 : Outport  Port=4  VectorParamsAs1DForOutWhenUnconnected=off
  out_5 : Outport  Port=5  VectorParamsAs1DForOutWhenUnconnected=off
  out_6 : Outport  Port=6  VectorParamsAs1DForOutWhenUnconnected=off
  out_7 : Outport  Port=7  VectorParamsAs1DForOutWhenUnconnected=off
  out_8 : Outport  Port=8  VectorParamsAs1DForOutWhenUnconnected=off
  out_9 : Outport  Port=9  VectorParamsAs1DForOutWhenUnconnected=off
  wires:
  Delay4/1 -> Line buffer/1, out_3/1
  channel_in/1 -> out_1/1, Delay1/1
  Delay1/1 -> out_2/1, Delay4/1
  Delay3/1 -> out_8/1, Delay6/1
  Delay5/1 -> Line buffer1/1, out_6/1
  Delay6/1 -> out_9/1
  Line buffer/1 -> out_4/1, Delay2/1
  Line buffer1/1 -> out_7/1, Delay3/1
  Delay2/1 -> out_5/1, Delay5/1

== system sobelFilter2024a/sqrt_threshold2/Subsystem2/slicer ==
  channel_in : Inport
  Delay{1..6} (6 alike) : Delay  DelayLength=1  InitialCondition=0
  Line buffer : Delay  DelayLength=R-2  InitialCondition=0
  Line buffer1 : Delay  DelayLength=R-2  InitialCondition=0
  out_1 : Outport  VectorParamsAs1DForOutWhenUnconnected=off
  out_2 : Outport  Port=2  VectorParamsAs1DForOutWhenUnconnected=off
  out_3 : Outport  Port=3  VectorParamsAs1DForOutWhenUnconnected=off
  out_4 : Outport  Port=4  VectorParamsAs1DForOutWhenUnconnected=off
  out_5 : Outport  Port=5  VectorParamsAs1DForOutWhenUnconnected=off
  out_6 : Outport  Port=6  VectorParamsAs1DForOutWhenUnconnected=off
  out_7 : Outport  Port=7  VectorParamsAs1DForOutWhenUnconnected=off
  out_8 : Outport  Port=8  VectorParamsAs1DForOutWhenUnconnected=off
  out_9 : Outport  Port=9  VectorParamsAs1DForOutWhenUnconnected=off
  wires:
  Delay4/1 -> Line buffer/1, out_3/1
  channel_in/1 -> out_1/1, Delay1/1
  Delay1/1 -> out_2/1, Delay4/1
  Delay3/1 -> out_8/1, Delay6/1
  Delay5/1 -> Line buffer1/1, out_6/1
  Delay6/1 -> out_9/1
  Line buffer/1 -> out_4/1, Delay2/1
  Line buffer1/1 -> out_7/1, Delay3/1
  Delay2/1 -> out_5/1, Delay5/1

== system sobelFilter2024a/sqrt_threshold2/Subsystem2/slicer1 ==
  channel_in : Inport
  Delay{1..6} (6 alike) : Delay  DelayLength=1  InitialCondition=0
  Line buffer : Delay  DelayLength=R-2  InitialCondition=0
  Line buffer1 : Delay  DelayLength=R-2  InitialCondition=0
  out_1 : Outport  VectorParamsAs1DForOutWhenUnconnected=off
  out_2 : Outport  Port=2  VectorParamsAs1DForOutWhenUnconnected=off
  out_3 : Outport  Port=3  VectorParamsAs1DForOutWhenUnconnected=off
  out_4 : Outport  Port=4  VectorParamsAs1DForOutWhenUnconnected=off
  out_5 : Outport  Port=5  VectorParamsAs1DForOutWhenUnconnected=off
  out_6 : Outport  Port=6  VectorParamsAs1DForOutWhenUnconnected=off
  out_7 : Outport  Port=7  VectorParamsAs1DForOutWhenUnconnected=off
  out_8 : Outport  Port=8  VectorParamsAs1DForOutWhenUnconnected=off
  out_9 : Outport  Port=9  VectorParamsAs1DForOutWhenUnconnected=off
  wires:
  Delay4/1 -> Line buffer/1, out_3/1
  channel_in/1 -> out_1/1, Delay1/1
  Delay1/1 -> out_2/1, Delay4/1
  Delay3/1 -> out_8/1, Delay6/1
  Delay5/1 -> Line buffer1/1, out_6/1
  Delay6/1 -> out_9/1
  Line buffer/1 -> out_4/1, Delay2/1
  Line buffer1/1 -> out_7/1, Delay3/1
  Delay2/1 -> out_5/1, Delay5/1

== system sobelFilter2024a/conv_core/gaussian_conv_core/Subsystem1/slicer ==
  channel_in : Inport
  Delay{1..6} (6 alike) : Delay  DelayLength=1  InitialCondition=0
  Line buffer : Delay  DelayLength=R-2  InitialCondition=0
  Line buffer1 : Delay  DelayLength=R-2  InitialCondition=0
  out_1 : Outport  VectorParamsAs1DForOutWhenUnconnected=off
  out_2 : Outport  Port=2  VectorParamsAs1DForOutWhenUnconnected=off
  out_3 : Outport  Port=3  VectorParamsAs1DForOutWhenUnconnected=off
  out_4 : Outport  Port=4  VectorParamsAs1DForOutWhenUnconnected=off
  out_5 : Outport  Port=5  VectorParamsAs1DForOutWhenUnconnected=off
  out_6 : Outport  Port=6  VectorParamsAs1DForOutWhenUnconnected=off
  out_7 : Outport  Port=7  VectorParamsAs1DForOutWhenUnconnected=off
  out_8 : Outport  Port=8  VectorParamsAs1DForOutWhenUnconnected=off
  out_9 : Outport  Port=9  VectorParamsAs1DForOutWhenUnconnected=off
  wires:
  Delay4/1 -> Line buffer/1, out_3/1
  channel_in/1 -> out_1/1, Delay1/1
  Delay1/1 -> out_2/1, Delay4/1
  Delay3/1 -> out_8/1, Delay6/1
  Delay5/1 -> Line buffer1/1, out_6/1
  Delay6/1 -> out_9/1
  Line buffer/1 -> out_4/1, Delay2/1
  Line buffer1/1 -> out_7/1, Delay3/1
  Delay2/1 -> out_5/1, Delay5/1

== system sobelFilter2024a/conv_core/sobel_horz_conv_core/Subsystem1/slicer ==
  channel_in : Inport
  Delay{1..6} (6 alike) : Delay  DelayLength=1  InitialCondition=0
  Line buffer : Delay  DelayLength=R-2  InitialCondition=0
  Line buffer1 : Delay  DelayLength=R-2  InitialCondition=0
  out_1 : Outport  VectorParamsAs1DForOutWhenUnconnected=off
  out_2 : Outport  Port=2  VectorParamsAs1DForOutWhenUnconnected=off
  out_3 : Outport  Port=3  VectorParamsAs1DForOutWhenUnconnected=off
  out_4 : Outport  Port=4  VectorParamsAs1DForOutWhenUnconnected=off
  out_5 : Outport  Port=5  VectorParamsAs1DForOutWhenUnconnected=off
  out_6 : Outport  Port=6  VectorParamsAs1DForOutWhenUnconnected=off
  out_7 : Outport  Port=7  VectorParamsAs1DForOutWhenUnconnected=off
  out_8 : Outport  Port=8  VectorParamsAs1DForOutWhenUnconnected=off
  out_9 : Outport  Port=9  VectorParamsAs1DForOutWhenUnconnected=off
  wires:
  Delay4/1 -> Line buffer/1, out_3/1
  channel_in/1 -> out_1/1, Delay1/1
  Delay1/1 -> out_2/1, Delay4/1
  Delay3/1 -> out_8/1, Delay6/1
  Delay5/1 -> Line buffer1/1, out_6/1
  Delay6/1 -> out_9/1
  Line buffer/1 -> out_4/1, Delay2/1
  Line buffer1/1 -> out_7/1, Delay3/1
  Delay2/1 -> out_5/1, Delay5/1

== system sobelFilter2024a/conv_core/sobel_horz_conv_core_alt/Subsystem1/slicer ==
  channel_in : Inport
  Delay{1..6} (6 alike) : Delay  DelayLength=1  InitialCondition=0
  Line buffer : Delay  DelayLength=R-2  InitialCondition=0
  Line buffer1 : Delay  DelayLength=R-2  InitialCondition=0
  out_1 : Outport  VectorParamsAs1DForOutWhenUnconnected=off
  out_2 : Outport  Port=2  VectorParamsAs1DForOutWhenUnconnected=off
  out_3 : Outport  Port=3  VectorParamsAs1DForOutWhenUnconnected=off
  out_4 : Outport  Port=4  VectorParamsAs1DForOutWhenUnconnected=off
  out_5 : Outport  Port=5  VectorParamsAs1DForOutWhenUnconnected=off
  out_6 : Outport  Port=6  VectorParamsAs1DForOutWhenUnconnected=off
  out_7 : Outport  Port=7  VectorParamsAs1DForOutWhenUnconnected=off
  out_8 : Outport  Port=8  VectorParamsAs1DForOutWhenUnconnected=off
  out_9 : Outport  Port=9  VectorParamsAs1DForOutWhenUnconnected=off
  wires:
  Delay4/1 -> Line buffer/1, out_3/1
  channel_in/1 -> out_1/1, Delay1/1
  Delay1/1 -> out_2/1, Delay4/1
  Delay3/1 -> out_8/1, Delay6/1
  Delay5/1 -> Line buffer1/1, out_6/1
  Delay6/1 -> out_9/1
  Line buffer/1 -> out_4/1, Delay2/1
  Line buffer1/1 -> out_7/1, Delay3/1
  Delay2/1 -> out_5/1, Delay5/1

== system sobelFilter2024a/conv_core/sobel_vert_conv_core/Subsystem1/slicer ==
  channel_in : Inport
  Delay{1..6} (6 alike) : Delay  DelayLength=1  InitialCondition=0
  Line buffer : Delay  DelayLength=R-2  InitialCondition=0
  Line buffer1 : Delay  DelayLength=R-2  InitialCondition=0
  out_1 : Outport  VectorParamsAs1DForOutWhenUnconnected=off
  out_2 : Outport  Port=2  VectorParamsAs1DForOutWhenUnconnected=off
  out_3 : Outport  Port=3  VectorParamsAs1DForOutWhenUnconnected=off
  out_4 : Outport  Port=4  VectorParamsAs1DForOutWhenUnconnected=off
  out_5 : Outport  Port=5  VectorParamsAs1DForOutWhenUnconnected=off
  out_6 : Outport  Port=6  VectorParamsAs1DForOutWhenUnconnected=off
  out_7 : Outport  Port=7  VectorParamsAs1DForOutWhenUnconnected=off
  out_8 : Outport  Port=8  VectorParamsAs1DForOutWhenUnconnected=off
  out_9 : Outport  Port=9  VectorParamsAs1DForOutWhenUnconnected=off
  wires:
  Delay4/1 -> Line buffer/1, out_3/1
  channel_in/1 -> out_1/1, Delay1/1
  Delay1/1 -> out_2/1, Delay4/1
  Delay3/1 -> out_8/1, Delay6/1
  Delay5/1 -> Line buffer1/1, out_6/1
  Delay6/1 -> out_9/1
  Line buffer/1 -> out_4/1, Delay2/1
  Line buffer1/1 -> out_7/1, Delay3/1
  Delay2/1 -> out_5/1, Delay5/1

== system sobelFilter2024a/conv_core/sobel_vert_conv_core_alt/Subsystem1/slicer ==
  channel_in : Inport
  Delay{1..6} (6 alike) : Delay  DelayLength=1  InitialCondition=0
  Line buffer : Delay  DelayLength=R-2  InitialCondition=0
  Line buffer1 : Delay  DelayLength=R-2  InitialCondition=0
  out_1 : Outport  VectorParamsAs1DForOutWhenUnconnected=off
  out_2 : Outport  Port=2  VectorParamsAs1DForOutWhenUnconnected=off
  out_3 : Outport  Port=3  VectorParamsAs1DForOutWhenUnconnected=off
  out_4 : Outport  Port=4  VectorParamsAs1DForOutWhenUnconnected=off
  out_5 : Outport  Port=5  VectorParamsAs1DForOutWhenUnconnected=off
  out_6 : Outport  Port=6  VectorParamsAs1DForOutWhenUnconnected=off
  out_7 : Outport  Port=7  VectorParamsAs1DForOutWhenUnconnected=off
  out_8 : Outport  Port=8  VectorParamsAs1DForOutWhenUnconnected=off
  out_9 : Outport  Port=9  VectorParamsAs1DForOutWhenUnconnected=off
  wires:
  Delay4/1 -> Line buffer/1, out_3/1
  channel_in/1 -> out_1/1, Delay1/1
  Delay1/1 -> out_2/1, Delay4/1
  Delay3/1 -> out_8/1, Delay6/1
  Delay5/1 -> Line buffer1/1, out_6/1
  Delay6/1 -> out_9/1
  Line buffer/1 -> out_4/1, Delay2/1
  Line buffer1/1 -> out_7/1, Delay3/1
  Delay2/1 -> out_5/1, Delay5/1

== system sobelFilter2024a/conv_core/sqrt_threshold/Subsystem2/slicer ==
  channel_in : Inport
  Delay{1..6} (6 alike) : Delay  DelayLength=1  InitialCondition=0
  Line buffer : Delay  DelayLength=R-2  InitialCondition=0
  Line buffer1 : Delay  DelayLength=R-2  InitialCondition=0
  out_1 : Outport  VectorParamsAs1DForOutWhenUnconnected=off
  out_2 : Outport  Port=2  VectorParamsAs1DForOutWhenUnconnected=off
  out_3 : Outport  Port=3  VectorParamsAs1DForOutWhenUnconnected=off
  out_4 : Outport  Port=4  VectorParamsAs1DForOutWhenUnconnected=off
  out_5 : Outport  Port=5  VectorParamsAs1DForOutWhenUnconnected=off
  out_6 : Outport  Port=6  VectorParamsAs1DForOutWhenUnconnected=off
  out_7 : Outport  Port=7  VectorParamsAs1DForOutWhenUnconnected=off
  out_8 : Outport  Port=8  VectorParamsAs1DForOutWhenUnconnected=off
  out_9 : Outport  Port=9  VectorParamsAs1DForOutWhenUnconnected=off
  wires:
  Delay4/1 -> Line buffer/1, out_3/1
  channel_in/1 -> out_1/1, Delay1/1
  Delay1/1 -> out_2/1, Delay4/1
  Delay3/1 -> out_8/1, Delay6/1
  Delay5/1 -> Line buffer1/1, out_6/1
  Delay6/1 -> out_9/1
  Line buffer/1 -> out_4/1, Delay2/1
  Line buffer1/1 -> out_7/1, Delay3/1
  Delay2/1 -> out_5/1, Delay5/1

== system sobelFilter2024a/conv_core/sqrt_threshold/Subsystem2/slicer1 ==
  channel_in : Inport
  Delay{1..6} (6 alike) : Delay  DelayLength=1  InitialCondition=0
  Line buffer : Delay  DelayLength=R-2  InitialCondition=0
  Line buffer1 : Delay  DelayLength=R-2  InitialCondition=0
  out_1 : Outport  VectorParamsAs1DForOutWhenUnconnected=off
  out_2 : Outport  Port=2  VectorParamsAs1DForOutWhenUnconnected=off
  out_3 : Outport  Port=3  VectorParamsAs1DForOutWhenUnconnected=off
  out_4 : Outport  Port=4  VectorParamsAs1DForOutWhenUnconnected=off
  out_5 : Outport  Port=5  VectorParamsAs1DForOutWhenUnconnected=off
  out_6 : Outport  Port=6  VectorParamsAs1DForOutWhenUnconnected=off
  out_7 : Outport  Port=7  VectorParamsAs1DForOutWhenUnconnected=off
  out_8 : Outport  Port=8  VectorParamsAs1DForOutWhenUnconnected=off
  out_9 : Outport  Port=9  VectorParamsAs1DForOutWhenUnconnected=off
  wires:
  Delay4/1 -> Line buffer/1, out_3/1
  channel_in/1 -> out_1/1, Delay1/1
  Delay1/1 -> out_2/1, Delay4/1
  Delay3/1 -> out_8/1, Delay6/1
  Delay5/1 -> Line buffer1/1, out_6/1
  Delay6/1 -> out_9/1
  Line buffer/1 -> out_4/1, Delay2/1
  Line buffer1/1 -> out_7/1, Delay3/1
  Delay2/1 -> out_5/1, Delay5/1

== system sobelFilter2024a/conv_core/sqrt_threshold1/Subsystem2/slicer ==
  channel_in : Inport
  Delay{1..6} (6 alike) : Delay  DelayLength=1  InitialCondition=0
  Line buffer : Delay  DelayLength=R-2  InitialCondition=0
  Line buffer1 : Delay  DelayLength=R-2  InitialCondition=0
  out_1 : Outport  VectorParamsAs1DForOutWhenUnconnected=off
  out_2 : Outport  Port=2  VectorParamsAs1DForOutWhenUnconnected=off
  out_3 : Outport  Port=3  VectorParamsAs1DForOutWhenUnconnected=off
  out_4 : Outport  Port=4  VectorParamsAs1DForOutWhenUnconnected=off
  out_5 : Outport  Port=5  VectorParamsAs1DForOutWhenUnconnected=off
  out_6 : Outport  Port=6  VectorParamsAs1DForOutWhenUnconnected=off
  out_7 : Outport  Port=7  VectorParamsAs1DForOutWhenUnconnected=off
  out_8 : Outport  Port=8  VectorParamsAs1DForOutWhenUnconnected=off
  out_9 : Outport  Port=9  VectorParamsAs1DForOutWhenUnconnected=off
  wires:
  Delay4/1 -> Line buffer/1, out_3/1
  channel_in/1 -> out_1/1, Delay1/1
  Delay1/1 -> out_2/1, Delay4/1
  Delay3/1 -> out_8/1, Delay6/1
  Delay5/1 -> Line buffer1/1, out_6/1
  Delay6/1 -> out_9/1
  Line buffer/1 -> out_4/1, Delay2/1
  Line buffer1/1 -> out_7/1, Delay3/1
  Delay2/1 -> out_5/1, Delay5/1

== system sobelFilter2024a/conv_core/sqrt_threshold1/Subsystem2/slicer1 ==
  channel_in : Inport
  Delay{1..6} (6 alike) : Delay  DelayLength=1  InitialCondition=0
  Line buffer : Delay  DelayLength=R-2  InitialCondition=0
  Line buffer1 : Delay  DelayLength=R-2  InitialCondition=0
  out_1 : Outport  VectorParamsAs1DForOutWhenUnconnected=off
  out_2 : Outport  Port=2  VectorParamsAs1DForOutWhenUnconnected=off
  out_3 : Outport  Port=3  VectorParamsAs1DForOutWhenUnconnected=off
  out_4 : Outport  Port=4  VectorParamsAs1DForOutWhenUnconnected=off
  out_5 : Outport  Port=5  VectorParamsAs1DForOutWhenUnconnected=off
  out_6 : Outport  Port=6  VectorParamsAs1DForOutWhenUnconnected=off
  out_7 : Outport  Port=7  VectorParamsAs1DForOutWhenUnconnected=off
  out_8 : Outport  Port=8  VectorParamsAs1DForOutWhenUnconnected=off
  out_9 : Outport  Port=9  VectorParamsAs1DForOutWhenUnconnected=off
  wires:
  Delay4/1 -> Line buffer/1, out_3/1
  channel_in/1 -> out_1/1, Delay1/1
  Delay1/1 -> out_2/1, Delay4/1
  Delay3/1 -> out_8/1, Delay6/1
  Delay5/1 -> Line buffer1/1, out_6/1
  Delay6/1 -> out_9/1
  Line buffer/1 -> out_4/1, Delay2/1
  Line buffer1/1 -> out_7/1, Delay3/1
  Delay2/1 -> out_5/1, Delay5/1

== system sobelFilter2024a/conv_core/sqrt_threshold2/Subsystem2/slicer ==
  channel_in : Inport
  Delay{1..6} (6 alike) : Delay  DelayLength=1  InitialCondition=0
  Line buffer : Delay  DelayLength=R-2  InitialCondition=0
  Line buffer1 : Delay  DelayLength=R-2  InitialCondition=0
  out_1 : Outport  VectorParamsAs1DForOutWhenUnconnected=off
  out_2 : Outport  Port=2  VectorParamsAs1DForOutWhenUnconnected=off
  out_3 : Outport  Port=3  VectorParamsAs1DForOutWhenUnconnected=off
  out_4 : Outport  Port=4  VectorParamsAs1DForOutWhenUnconnected=off
  out_5 : Outport  Port=5  VectorParamsAs1DForOutWhenUnconnected=off
  out_6 : Outport  Port=6  VectorParamsAs1DForOutWhenUnconnected=off
  out_7 : Outport  Port=7  VectorParamsAs1DForOutWhenUnconnected=off
  out_8 : Outport  Port=8  VectorParamsAs1DForOutWhenUnconnected=off
  out_9 : Outport  Port=9  VectorParamsAs1DForOutWhenUnconnected=off
  wires:
  Delay4/1 -> Line buffer/1, out_3/1
  channel_in/1 -> out_1/1, Delay1/1
  Delay1/1 -> out_2/1, Delay4/1
  Delay3/1 -> out_8/1, Delay6/1
  Delay5/1 -> Line buffer1/1, out_6/1
  Delay6/1 -> out_9/1
  Line buffer/1 -> out_4/1, Delay2/1
  Line buffer1/1 -> out_7/1, Delay3/1
  Delay2/1 -> out_5/1, Delay5/1

== system sobelFilter2024a/conv_core/sqrt_threshold2/Subsystem2/slicer1 ==
  channel_in : Inport
  Delay{1..6} (6 alike) : Delay  DelayLength=1  InitialCondition=0
  Line buffer : Delay  DelayLength=R-2  InitialCondition=0
  Line buffer1 : Delay  DelayLength=R-2  InitialCondition=0
  out_1 : Outport  VectorParamsAs1DForOutWhenUnconnected=off
  out_2 : Outport  Port=2  VectorParamsAs1DForOutWhenUnconnected=off
  out_3 : Outport  Port=3  VectorParamsAs1DForOutWhenUnconnected=off
  out_4 : Outport  Port=4  VectorParamsAs1DForOutWhenUnconnected=off
  out_5 : Outport  Port=5  VectorParamsAs1DForOutWhenUnconnected=off
  out_6 : Outport  Port=6  VectorParamsAs1DForOutWhenUnconnected=off
  out_7 : Outport  Port=7  VectorParamsAs1DForOutWhenUnconnected=off
  out_8 : Outport  Port=8  VectorParamsAs1DForOutWhenUnconnected=off
  out_9 : Outport  Port=9  VectorParamsAs1DForOutWhenUnconnected=off
  wires:
  Delay4/1 -> Line buffer/1, out_3/1
  channel_in/1 -> out_1/1, Delay1/1
  Delay1/1 -> out_2/1, Delay4/1
  Delay3/1 -> out_8/1, Delay6/1
  Delay5/1 -> Line buffer1/1, out_6/1
  Delay6/1 -> out_9/1
  Line buffer/1 -> out_4/1, Delay2/1
  Line buffer1/1 -> out_7/1, Delay3/1
  Delay2/1 -> out_5/1, Delay5/1
